simulink model "AO"  (R2018a)
settings: Solver=FixedStepAuto  StartTime=0.0  StopTime=10.0  RelTol=1e-3  EnableMultiTasking=on
libraries: arduinolib x4
settings Model: ExtModeTrigDuration=2  Creator=yupuic  LastModifiedBy=yupuic
settings DataIOCC: ExternalInput=[t in1]  InitialState=0
settings OptimizationCC: EnhancedBackFolding=on  PassReuseOutputArgsThreshold=0  MaxStackSize=64  OptimizeBlockOrder=speed  DifferentSizesBufferReuse=on  OptimizationCustomize=off
settings DebuggingCC: ParameterTunabilityLossMsg=error
settings HardwareCC: ProdBitPerInt=16  ProdBitPerPointer=16  ProdBitPerSizeT=16  ProdBitPerPtrDiffT=16  ProdLargestAtomicFloat=None  ProdWordSize=8  ProdHWDeviceType=Atmel->AVR  UseEmbeddedCoderFeatures=off  UseSimulinkCoderFeatures=off
settings SFSimCC: MATLABDynamicMemAlloc=off
settings RTWCC: SystemTargetFile=ert.tlc  HardwareBoard=Arduino Uno  TLCOptions=-aInlineSetEventsForThisBaseRateFcn=TLC_FALSE -aSuppressMultiTaskScheduler=TLC_FALSE -aRateBasedStepFcn=1  TemplateMakefile=ert_default_tmf  GenerateReport=on  Toolchain=Arduino AVR  BuildConfiguration=Faster Runs  LaunchReport=on
settings CodeAppCC: ForceParamTrailComments=on  OperatorAnnotations=on
settings ERTTargetCC: ERTCustomFileBanners=off  SupportContinuousTime=on  SupportNonInlinedSFcns=on  RemoveResetFunc=off  SupportVariableSizeSignals=on  ModelStepFunctionPrototypeControlCompliant=off

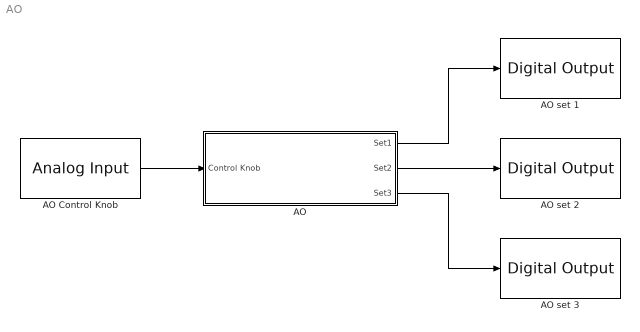
== system AO ==
  AO : Subsystem
  AO Control Knob : arduinolib/Analog Input  pinNumber=0  ReadResultsOnly=off  ConversionTriggerSource=Software  ExternalTriggerType=uint32(0)  OutputDataType=uint16  EnableConversionCompleteNotify=off  EnableOuputStatus=off  SampleTime=1  blockPlatform=arduino
  AO set 1 : arduinolib/Digital Output  pinNumber=5  blockPlatform=arduino
  AO set 2 : arduinolib/Digital Output  pinNumber=6  blockPlatform=arduino
  AO set 3 : arduinolib/Digital Output  pinNumber=7  blockPlatform=arduino
  wires:
  AO/1(Set1) -> AO set 1/1
  AO/3(Set3) -> AO set 3/1
  AO Control Knob/1 -> AO/1(Control Knob)
  AO/2(Set2) -> AO set 2/1

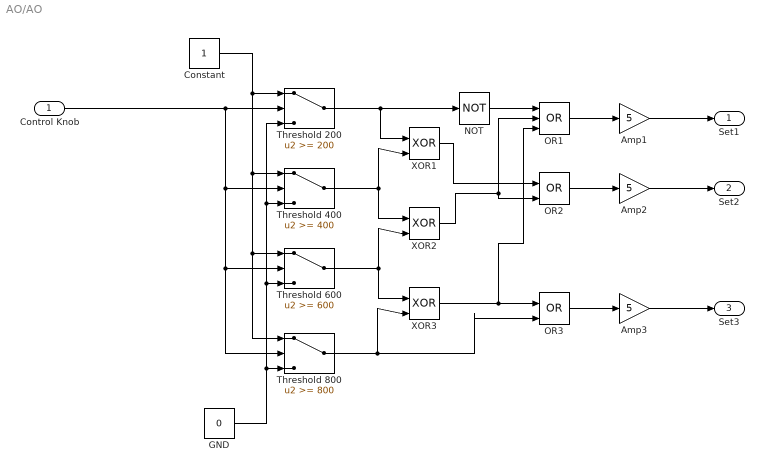
== system AO/AO ==
  Control Knob : Inport
  Amp1 : Gain  Gain=5
  Amp2 : Gain  Gain=5
  Amp3 : Gain  Gain=5
  Constant : Constant
  "GND " : Constant  Value=0
  "NOT " : Logic  Operator=NOT  Inputs=1  IconShape=distinctive  AllPortsSameDT=off  OutDataTypeStr=boolean
  OR1 : Logic  Operator=OR  Inputs=3  IconShape=distinctive  AllPortsSameDT=off  OutDataTypeStr=boolean
  OR2 : Logic  Operator=OR  IconShape=distinctive  AllPortsSameDT=off  OutDataTypeStr=boolean
  OR3 : Logic  Operator=OR  IconShape=distinctive  AllPortsSameDT=off  OutDataTypeStr=boolean
  Threshold 200 : Switch  Threshold=200
  Threshold 400 : Switch  Threshold=400
  Threshold 600 : Switch  Threshold=600
  Threshold 800 : Switch  Threshold=800
  XOR1 : Logic  Operator=XOR  IconShape=distinctive  AllPortsSameDT=off  OutDataTypeStr=boolean
  XOR2 : Logic  Operator=XOR  IconShape=distinctive  AllPortsSameDT=off  OutDataTypeStr=boolean
  XOR3 : Logic  Operator=XOR  IconShape=distinctive  AllPortsSameDT=off  OutDataTypeStr=boolean
  Set1 : Outport
  Set2 : Outport  Port=2
  Set3 : Outport  Port=3
  wires:
  XOR2/1 -> OR1/2, OR2/2
  Threshold 600/1 -> XOR2/2, XOR3/1
  Threshold 200/1 -> "NOT "/1, XOR1/1
  "GND "/1 -> Threshold 200/3, Threshold 400/3, Threshold 600/3, Threshold 800/3
  Threshold 800/1 -> OR3/2, XOR3/2
  Control Knob/1 -> Threshold 400/2, Threshold 600/2, Threshold 800/2, Threshold 200/2
  Threshold 400/1 -> XOR1/2, XOR2/1
  XOR3/1 -> OR1/3, OR3/1
  Constant/1 -> Threshold 800/1, Threshold 600/1, Threshold 400/1, Threshold 200/1
  "NOT "/1 -> OR1/1
  XOR1/1 -> OR2/1
  OR1/1 -> Amp1/1
  Amp1/1 -> Set1/1
  OR2/1 -> Amp2/1
  Amp2/1 -> Set2/1
  OR3/1 -> Amp3/1
  Amp3/1 -> Set3/1
